simulink model "Implantation_Cmd_LQ"  (R2018b)
settings: Solver=ode1  StartTime=0.0  StopTime=15  FixedStep=Te1  RelTol=1e-3  EnableMultiTasking=on
values from neighbouring files (symbols this model uses):
  K_lq = []    [InitCommande_Aero.m]
  Kw = Ka(1)    [InitCommande_Aero.m]    (also in apoio (1).m; matlab_variables.mat = 0.240350108962)
  Kz = Ka(2)    [InitCommande_Aero.m]    (also in apoio (1).m; matlab_variables.mat = 4.57892915652)
  M_lq = []    [InitCommande_Aero.m]
  Te1 = 0.002    [InitCommande_Aero.m]    (also in apoio (1).m; matlab_variables.mat)
  Te2 = 0.02    [InitCommande_Aero.m]
libraries: quanser_aero x1, simulink_extras x1
settings Model: SimulationMode=external  ExtModeTrigDuration=50000  Creator=MLevis  LastModifiedBy=Rodriguez
settings SolverCC: PositivePriorityOrder=on
settings DataIOCC: SaveFormat=Array  DSMLogging=off
settings OptimizationCC: LifeSpan=inf
settings DebuggingCC: SolverPrmCheckMsg=warning  SFUnexpectedBacktrackingDiag=warning  SFNoUnconditionalDefaultTransitionDiag=warning  SFExecutionAtInitializationDiag=none
settings HardwareCC: ProdBitPerPointer=32  ProdBitPerSizeT=32  ProdBitPerPtrDiffT=32  ProdLargestAtomicFloat=None  ProdIntDivRoundTo=Undefined  ProdEndianess=Unspecified  ProdWordSize=32  ProdHWDeviceType=32-bit Generic
settings ModelReferenceCC: PropagateSignalLabelsOutOfModel=off
settings SFSimCC: SimUseLocalCustomCode=off
settings RTWCC: SystemTargetFile=quarc_win64.tlc  TemplateMakefile=quarc_default_tmf  Description=QUARC Win64 Target  RTWUseLocalCustomCode=off
settings CodeAppCC: StateflowObjectComments=on
settings STFCustomTargetCC: TargetPreCompLibLocation=C:\PROGRA~3\QUARC\lib\2018b\win64\release  ConcurrentExecutionCompliant=on  GeneratePreprocessorConditionals=Disable all  GRTInterface=on  SystemTargetFile=quarc_win64.tlc
settings GRTTargetCC: TargetPreCompLibLocation=C:\PROGRA~3\QUARC\lib\2018b\win64\release  TargetLangStandard=C89/C90 (ANSI)  ParMdlRefBuildCompliant=off  CompOptLevelCompliant=off  GeneratePreprocessorConditionals=Disable all  CombineOutputUpdateFcns=off  MatFileLogging=off  CPPClassGenCompliant=off  GRTInterface=on  UseToolchainInfoCompliant=off  ExtMode=on  ExtModeMexFile=quarc_comm
settings ConfigComp: CovMetricSettings=dw  CovHtmlReporting=on  CovSaveCumulativeToWorkspaceVar=on  CovSaveSingleToWorkspaceVar=on  CovExternalEMLEnable=off  CovSFcnEnable=off

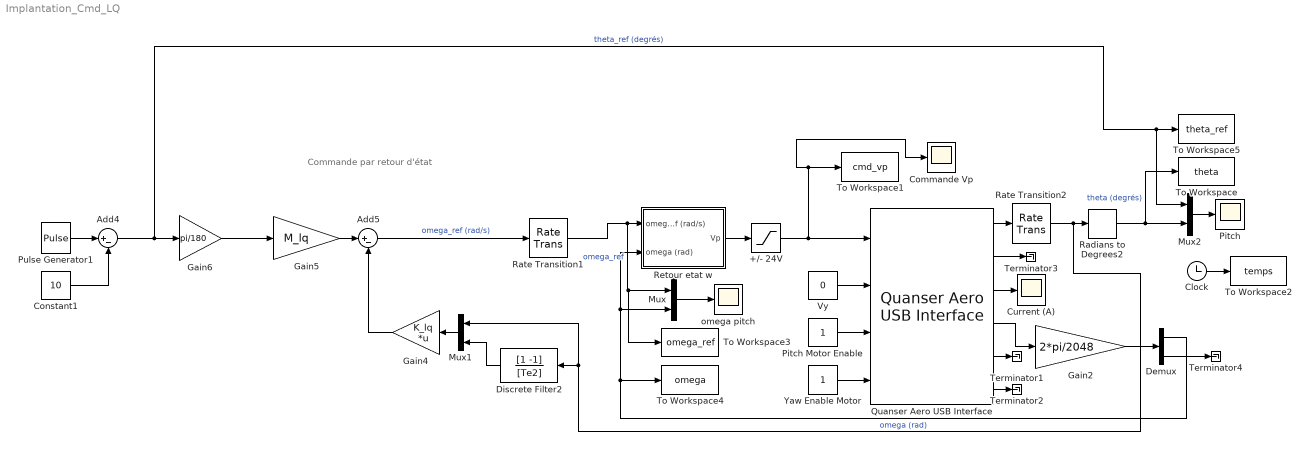
== system Implantation_Cmd_LQ ==
  note: Commande par retour d'état
  +/- 24V : Saturate  UpperLimit=24  LowerLimit=-24
  Add4 : Sum  Inputs=|+-
  Add5 : Sum  Inputs=|+-
  Clock : Clock
  Commande Vp : Scope
  Constant1 : Constant  Value=10
  Current (A) : Scope
  Demux : Demux  Outputs=2
  Discrete Filter2 : DiscreteFilter  Numerator=[1 -1]  Denominator=[Te2]  SampleTime=Te2
  Gain2 : Gain  Gain=2*pi/2048
  Gain4 : Gain  Gain=K_lq  Multiplication=Matrix(K*u)
  Gain5 : Gain  Gain=M_lq
  Gain6 : Gain  Gain=pi/180
  Mux : Mux  Inputs=2
  Mux1 : Mux  Inputs=2
  Mux2 : Mux  Inputs=2
  Pitch : Scope
  Pitch Motor Enable : Constant
  Pulse Generator1 : DiscretePulseGenerator  Amplitude=20  Period=ceil(20/Te2)  PulseWidth=ceil(10/Te2)  SampleTime=Te2
  Quanser Aero USB Interface : quanser_aero/Quanser Aero USB Interface  SystemSampleTime=-1
  Radians to Degrees2 : simulink_extras/Transformations/Radians to Degrees
  Rate Transition1 : RateTransition  OutPortSampleTime=Te1
  Rate Transition2 : RateTransition  OutPortSampleTime=Te2
  Retour etat w : Subsystem
  Terminator{1..4} (4 alike) : Terminator
  To Workspace : ToWorkspace  VariableName=theta  SampleTime=-1
      settings: Save2DSignal=2-D array (concatenate along first dimension)
  To Workspace1 : ToWorkspace  VariableName=cmd_vp  SampleTime=-1
      settings: Save2DSignal=2-D array (concatenate along first dimension)
  To Workspace2 : ToWorkspace  VariableName=temps  SampleTime=-1
      settings: Save2DSignal=2-D array (concatenate along first dimension)
  To Workspace3 : ToWorkspace  VariableName=omega_ref  SampleTime=-1
      settings: Save2DSignal=2-D array (concatenate along first dimension)
  To Workspace4 : ToWorkspace  VariableName=omega  SampleTime=-1
      settings: Save2DSignal=2-D array (concatenate along first dimension)
  To Workspace5 : ToWorkspace  VariableName=theta_ref  SampleTime=-1
      settings: Save2DSignal=2-D array (concatenate along first dimension)
  Vy : Constant  Value=0
  Yaw Enable Motor : Constant
  omega pitch : Scope
  wires:
  Pitch Motor Enable/1 -> Quanser Aero USB Interface/3
  Yaw Enable Motor/1 -> Quanser Aero USB Interface/4
  +/- 24V/1 -> Quanser Aero USB Interface/1, Commande Vp/1, To Workspace1/1
  Quanser Aero USB Interface/3 -> Current (A)/1
  Quanser Aero USB Interface/1 -> Rate Transition2/1
  Quanser Aero USB Interface/4 -> Gain2/1
  Quanser Aero USB Interface/5 -> Terminator1/1
  Quanser Aero USB Interface/6 -> Terminator2/1
  Vy/1 -> Quanser Aero USB Interface/2
  Quanser Aero USB Interface/2 -> Terminator3/1
  Clock/1 -> To Workspace2/1
  Add5/1 -> Rate Transition1/1  "omega_ref (rad/s)"
  Gain2/1 -> Demux/1
  Demux/2 -> Terminator4/1
  Demux/1 -> Retour etat w/2(omega (rad)), Mux/2, To Workspace4/1  "omega (rad)"
  Gain5/1 -> Add5/1
  Gain4/1 -> Add5/2
  Pulse Generator1/1 -> Add4/1
  Constant1/1 -> Add4/2
  Gain6/1 -> Gain5/1
  Add4/1 -> Mux2/1, To Workspace5/1, Gain6/1  "theta_ref (degrés)"
  Mux1/1 -> Gain4/1
  Rate Transition2/1 -> Radians to Degrees2/1, Mux1/1, Discrete Filter2/1
  Rate Transition1/1 -> To Workspace3/1, Mux/1, Retour etat w/1(omega_ref (rad/s))  "omega_ref"
  Radians to Degrees2/1 -> Mux2/2, To Workspace/1  "theta (degrés)"
  Mux2/1 -> Pitch/1
  Retour etat w/1(Vp) -> +/- 24V/1
  Discrete Filter2/1 -> Mux1/2
  Mux/1 -> omega pitch/1

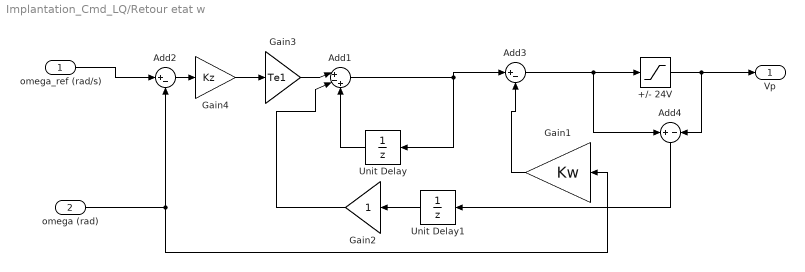
== system Implantation_Cmd_LQ/Retour etat w ==
  omega_ref (rad/s) : Inport
  omega (rad) : Inport  Port=2
  +/- 24V : Saturate  UpperLimit=24  LowerLimit=-24
  Add1 : Sum  Inputs=|+-+
  Add2 : Sum  Inputs=|+-
  Add3 : Sum  Inputs=|+-
  Add4 : Sum  Inputs=+-
  Gain1 : Gain  Gain=Kw
  Gain2 : Gain
  Gain3 : Gain  Gain=Te1
  Gain4 : Gain  Gain=Kz
  Unit Delay : UnitDelay  SampleTime=Te1
  Unit Delay1 : UnitDelay  SampleTime=Te1
  Vp : Outport
  wires:
  omega_ref (rad/s)/1 -> Add2/1
  Add2/1 -> Gain4/1
  omega (rad)/1 -> Add2/2, Gain1/1
  Gain1/1 -> Add3/2
  Add3/1 -> Add4/1, +/- 24V/1
  Gain3/1 -> Add1/1
  +/- 24V/1 -> Add4/2, Vp/1
  Gain4/1 -> Gain3/1
  Add1/1 -> Unit Delay/1, Add3/1
  Add4/1 -> Unit Delay1/1
  Unit Delay/1 -> Add1/3
  Gain2/1 -> Add1/2
  Unit Delay1/1 -> Gain2/1
